simulink model "CAS_MPPT_ESC"  (R2022a)
settings: Solver=VariableStepAuto  StartTime=0.0  StopTime=24  RelTol=1e-12
undefined symbols (not defined in the file or in its folder): sigbuilder_block
settings Model: PacingRate=0.400000  Creator=samso  LastModifiedBy=samso
settings OptimizationCC: BlockReduction=off  DefaultParameterBehavior=Inlined  BufferReuse=off

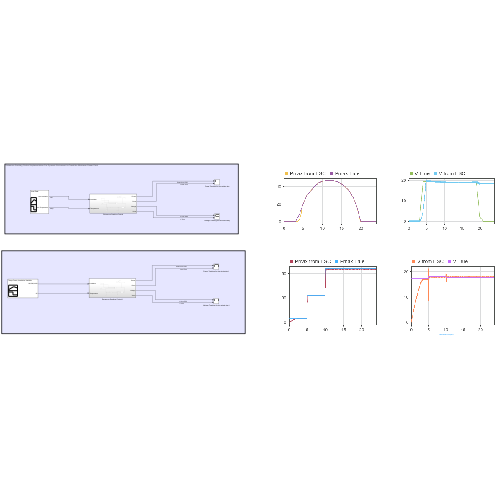
[thumbnail: Simulink's stored preview of the top-level diagram]
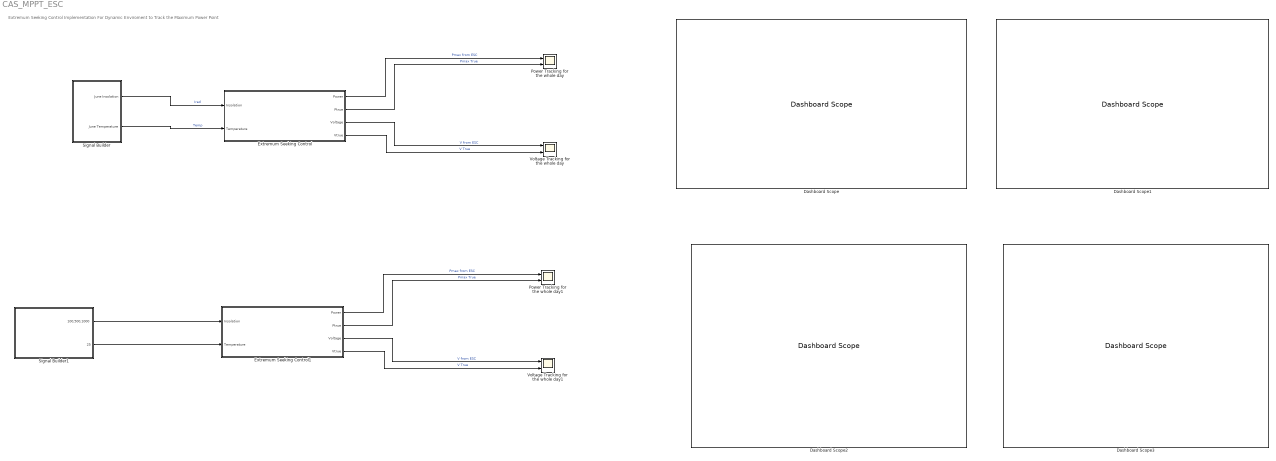
== system CAS_MPPT_ESC ==
  note: Extremum Seeking Control Implementation For Dynamic Enviroment to Track the Maximum Power Point
  Dashboard Scope{,1..3} (4 alike) : DashboardScope
  Extremum Seeking Control : Subsystem
  Extremum Seeking Control1 : Subsystem
  Power Tracking for the whole day : Scope  NumInputPorts=2
  Power Tracking for the whole day1 : Scope  NumInputPorts=2
  Signal Builder : Subsystem  Tag=STV Subsys  LoadFcn=sigbuilder_block('load');  StartFcn=sigbuilder_block('start');  StopFcn=sigbuilder_block('stop');  ClipboardFcn=sigbuilder_block('clipboard');  mask(Sigbuilder block){tuvar=[0:10]}
      mask help: Simulink:masks:SigbuilderBlock_MD
      mask init:
      | if ~strcmp(get_param(bdroot(gcbh),'SimulationStatus'),'stopped') tuvar = sigbuilder_block('maskInit'); end
      settings: CopyFcn=sigbuilder_block('copy');  DeleteFcn=sigbuilder_block('delete');  ModelCloseFcn=sigbuilder_block('modelClose');  PreSaveFcn=sigbuilder_block('preSave');  PauseFcn=sigbuilder_block('pause');  ContinueFcn=sigbuilder_block('continue');  NameChangeFcn=sigbuilder_block('namechange');  OpenFcn=sigbuilder_block('open',[437.25 199.5 386.25 399.75 ]);  CloseFcn=sigbuilder_block('close');
      mask Display: plot(0, 0, 100, 100,[2, 2, 32, 32, 2], [68, 8, 8, 68, 68],[32, 2], [38, 38], [32, 19, 2],[53, 60, 44], [32, 17, 17, 2],[16, 16, 31, 31]);txt = getActiveGroup(gcbh);text(2, 100, txt,'verticalAlignment', 'top');
  Signal Builder1 : Subsystem  Tag=STV Subsys  LoadFcn=sigbuilder_block('load');  StartFcn=sigbuilder_block('start');  StopFcn=sigbuilder_block('stop');  ClipboardFcn=sigbuilder_block('clipboard');  mask(Sigbuilder block){tuvar=[0:10]}
      mask help: Simulink:masks:SigbuilderBlock_MD
      mask init:
      | if ~strcmp(get_param(bdroot(gcbh),'SimulationStatus'),'stopped') tuvar = sigbuilder_block('maskInit'); end
      settings: CopyFcn=sigbuilder_block('copy');  DeleteFcn=sigbuilder_block('delete');  ModelCloseFcn=sigbuilder_block('modelClose');  PreSaveFcn=sigbuilder_block('preSave');  PauseFcn=sigbuilder_block('pause');  ContinueFcn=sigbuilder_block('continue');  NameChangeFcn=sigbuilder_block('namechange');  OpenFcn=sigbuilder_block('open',[0 36 1440 716.25 ]);  CloseFcn=sigbuilder_block('close');
      mask Display: plot(0, 0, 100, 100,[2, 2, 32, 32, 2], [68, 8, 8, 68, 68],[32, 2], [38, 38], [32, 19, 2],[53, 60, 44], [32, 17, 17, 2],[16, 16, 31, 31]);txt = getActiveGroup(gcbh);text(2, 100, txt,'verticalAlignment', 'top');
  Voltage Tracking for the whole day : Scope  NumInputPorts=2
  Voltage Tracking for the whole day1 : Scope  NumInputPorts=2
  wires:
  Extremum Seeking Control/1(Power) -> Power Tracking for the whole day/1  "Pmax from ESC"
  Extremum Seeking Control/2(Ptrue) -> Power Tracking for the whole day/2  "Pmax True"
  Extremum Seeking Control/3(Voltage) -> Voltage Tracking for the whole day/1  "V from ESC"
  Extremum Seeking Control/4(Vtrue) -> Voltage Tracking for the whole day/2  "V True"
  Signal Builder/1(June Insolation) -> Extremum Seeking Control/1(Insolation)  "Irad"
  Signal Builder/2(June Temperature) -> Extremum Seeking Control/2(Temperature)  "Temp"
  Extremum Seeking Control1/3(Voltage) -> Voltage Tracking for the whole day1/1  "V from ESC"
  Extremum Seeking Control1/1(Power) -> Power Tracking for the whole day1/1  "Pmax from ESC"
  Extremum Seeking Control1/4(Vtrue) -> Voltage Tracking for the whole day1/2  "V True"
  Extremum Seeking Control1/2(Ptrue) -> Power Tracking for the whole day1/2  "Pmax True"
  Signal Builder1/1(100,500,1000) -> Extremum Seeking Control1/1(Insolation)
  Signal Builder1/2(25) -> Extremum Seeking Control1/2(Temperature)

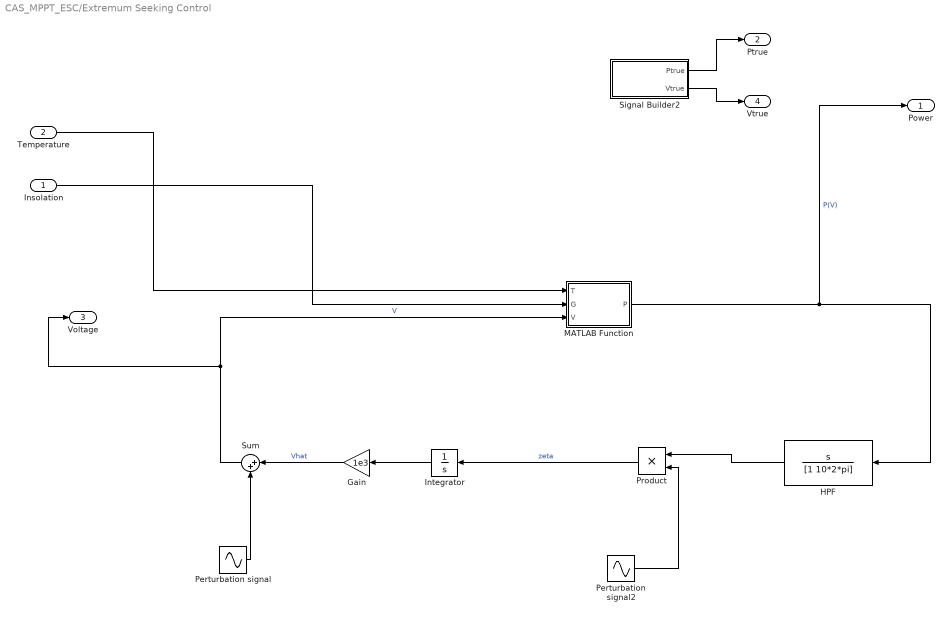
== system CAS_MPPT_ESC/Extremum Seeking Control ==
  Insolation : Inport
  Temperature : Inport  Port=2
  Gain : Gain  Gain=1e3
  HPF : TransferFcn  Numerator=[1 0]  Denominator=[1 10*2*pi]
  Integrator : Integrator
  MATLAB Function : MATLAB Function  TreatAsAtomicUnit=on
  Perturbation signal : Sin  Amplitude=0.2  Frequency=25*2*pi  SampleTime=0
  Perturbation signal2 : Sin  Amplitude=0.2  Frequency=25*2*pi  SampleTime=0
  Product : Product
  Signal Builder2 : Subsystem  Tag=STV Subsys  LoadFcn=sigbuilder_block('load');  StartFcn=sigbuilder_block('start');  StopFcn=sigbuilder_block('stop');  ClipboardFcn=sigbuilder_block('clipboard');  mask(Sigbuilder block){tuvar=[0:10]}
      mask help: Simulink:masks:SigbuilderBlock_MD
      mask init:
      | if ~strcmp(get_param(bdroot(gcbh),'SimulationStatus'),'stopped') tuvar = sigbuilder_block('maskInit'); end
      settings: CopyFcn=sigbuilder_block('copy');  DeleteFcn=sigbuilder_block('delete');  ModelCloseFcn=sigbuilder_block('modelClose');  PreSaveFcn=sigbuilder_block('preSave');  PauseFcn=sigbuilder_block('pause');  ContinueFcn=sigbuilder_block('continue');  NameChangeFcn=sigbuilder_block('namechange');  OpenFcn=sigbuilder_block('open',[6 36 1428 675.75 ]);  CloseFcn=sigbuilder_block('close');
      mask Display: plot(0, 0, 100, 100,[2, 2, 32, 32, 2], [68, 8, 8, 68, 68],[32, 2], [38, 38], [32, 19, 2],[53, 60, 44], [32, 17, 17, 2],[16, 16, 31, 31]);txt = getActiveGroup(gcbh);text(2, 100, txt,'verticalAlignment', 'top');
  Sum : Sum  Inputs=|++
  Power : Outport
  Ptrue : Outport  Port=2
  Voltage : Outport  Port=3
  Vtrue : Outport  Port=4
  wires:
  Product/1 -> Integrator/1  "zeta"
  Perturbation signal/1 -> Sum/2
  Integrator/1 -> Gain/1
  MATLAB Function/1(P) -> Power/1, HPF/1  "P(V)"
  HPF/1 -> Product/1
  Sum/1 -> Voltage/1, MATLAB Function/3(V)  "V"
  Perturbation signal2/1 -> Product/2
  Gain/1 -> Sum/1  "Vhat"
  Insolation/1 -> MATLAB Function/2(G)
  Temperature/1 -> MATLAB Function/1(T)
  Signal Builder2/1(Ptrue) -> Ptrue/1
  Signal Builder2/2(Vtrue) -> Vtrue/1

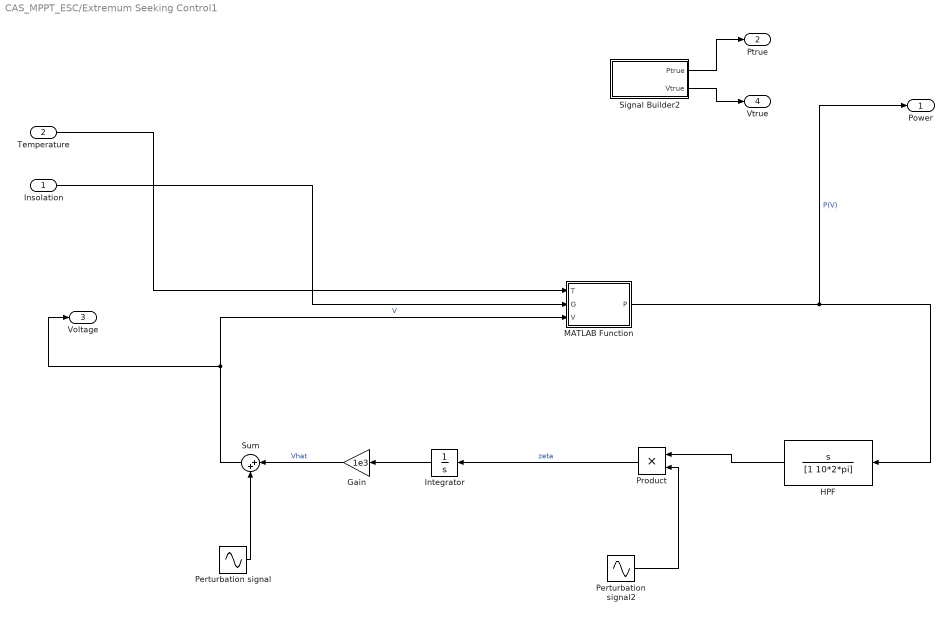
== system CAS_MPPT_ESC/Extremum Seeking Control1 ==
  Insolation : Inport
  Temperature : Inport  Port=2
  Gain : Gain  Gain=1e3
  HPF : TransferFcn  Numerator=[1 0]  Denominator=[1 10*2*pi]
  Integrator : Integrator
  MATLAB Function : MATLAB Function  TreatAsAtomicUnit=on
  Perturbation signal : Sin  Amplitude=0.2  Frequency=25*2*pi  SampleTime=0
  Perturbation signal2 : Sin  Amplitude=0.2  Frequency=25*2*pi  SampleTime=0
  Product : Product
  Signal Builder2 : Subsystem  Tag=STV Subsys  LoadFcn=sigbuilder_block('load');  StartFcn=sigbuilder_block('start');  StopFcn=sigbuilder_block('stop');  ClipboardFcn=sigbuilder_block('clipboard');  mask(Sigbuilder block){tuvar=[0:10]}
      mask help: Simulink:masks:SigbuilderBlock_MD
      mask init:
      | if ~strcmp(get_param(bdroot(gcbh),'SimulationStatus'),'stopped') tuvar = sigbuilder_block('maskInit'); end
      settings: CopyFcn=sigbuilder_block('copy');  DeleteFcn=sigbuilder_block('delete');  ModelCloseFcn=sigbuilder_block('modelClose');  PreSaveFcn=sigbuilder_block('preSave');  PauseFcn=sigbuilder_block('pause');  ContinueFcn=sigbuilder_block('continue');  NameChangeFcn=sigbuilder_block('namechange');  OpenFcn=sigbuilder_block('open',[6 36 1428 675.75 ]);  CloseFcn=sigbuilder_block('close');
      mask Display: plot(0, 0, 100, 100,[2, 2, 32, 32, 2], [68, 8, 8, 68, 68],[32, 2], [38, 38], [32, 19, 2],[53, 60, 44], [32, 17, 17, 2],[16, 16, 31, 31]);txt = getActiveGroup(gcbh);text(2, 100, txt,'verticalAlignment', 'top');
  Sum : Sum  Inputs=|++
  Power : Outport
  Ptrue : Outport  Port=2
  Voltage : Outport  Port=3
  Vtrue : Outport  Port=4
  wires:
  Product/1 -> Integrator/1  "zeta"
  Perturbation signal/1 -> Sum/2
  Integrator/1 -> Gain/1
  MATLAB Function/1(P) -> Power/1, HPF/1  "P(V)"
  HPF/1 -> Product/1
  Sum/1 -> Voltage/1, MATLAB Function/3(V)  "V"
  Perturbation signal2/1 -> Product/2
  Gain/1 -> Sum/1  "Vhat"
  Insolation/1 -> MATLAB Function/2(G)
  Temperature/1 -> MATLAB Function/1(T)
  Signal Builder2/2(Vtrue) -> Vtrue/1
  Signal Builder2/1(Ptrue) -> Ptrue/1

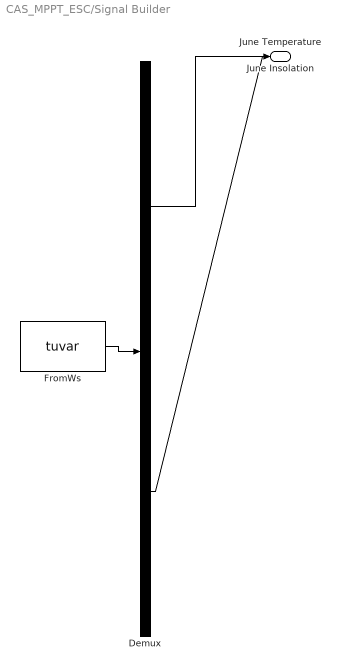
== system CAS_MPPT_ESC/Signal Builder ==
  Demux : Demux  Tag=STV Demux  Outputs=2
      settings: DisplayOption=none
  FromWs : FromWorkspace  Tag=STV FromWs  VariableName=tuvar
      SigBuilderData=|
      | common.afterFinalStr = 'Extrapolate'
      | common.sampleTime = 0
      | dataSet.timeRange = [0 24]
      | dataSet.name = 'June Data'
      | sbobj.Groups.Name = 'June Data'
      | sbobj.Groups.Signals(1).Name = 'June Insolation'
      | sbobj.Groups.Signals(1).XData = [0 1 2 3 4 5 6 7 8 9 10 11 12 13 14 15 16 17 18 19 20 21 22 24]
      | sbobj.Groups.Signals(1).YData = [0 0 0 0 139 297 435 500 576 630 662 676 679 679 657 624 577 509 409 255 5 0 0 0]
      | sbobj.Groups.Signals(2).Name = 'June Temperature'
      | sbobj.Groups.Signals(2).XData = [0 1 2 3 4 5 6 7 8 9 10 11 12 13 14 15 16 17 18 19 20 21 22 23 24]
      | sbobj.Groups.Signals(2).YData = [13.32 12.93 12.69 12.53 12.38 12.52 13.3 14.31 15.22 16.12 16.93 17.62 18.14 18.49 18.67 18.66 18.47 18.08 17.56 16.9 15.89 15 14.28 13.74 13.74]
      | sbobj.Groups.TimeRange = [0 24]
  June Insolation : Outport  Tag=STV Outport
  June Temperature : Outport  Tag=STV Outport  Port=2
  wires:
  FromWs/1 -> Demux/1
  Demux/1 -> June Insolation/1
  Demux/2 -> June Temperature/1

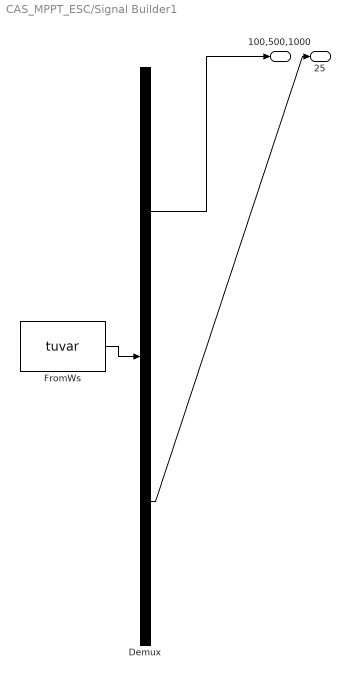
== system CAS_MPPT_ESC/Signal Builder1 ==
  Demux : Demux  Tag=STV Demux  Outputs=2
      settings: DisplayOption=none
  FromWs : FromWorkspace  Tag=STV FromWs  VariableName=tuvar
      SigBuilderData=|
      | common.afterFinalStr = 'Extrapolate'
      | common.sampleTime = 0
      | dataSet.timeRange = [0 24]
      | dataSet.name = 'Temp Const, Insolation Variable'
      | sbobj.Groups.Name = 'Temp Const, Insolation Variable'
      | sbobj.Groups.Signals(1).Name = '100,500,1000'
      | sbobj.Groups.Signals(1).XData = [0 5 5 10 10 24]
      | sbobj.Groups.Signals(1).YData = [100 100 500 500 1000 1000]
      | sbobj.Groups.Signals(2).Name = '25'
      | sbobj.Groups.Signals(2).XData = [0 24]
      | sbobj.Groups.Signals(2).YData = [25 25]
      | sbobj.Groups.TimeRange = [0 24]
  100,500,1000 : Outport  Tag=STV Outport
  25 : Outport  Tag=STV Outport  Port=2
  wires:
  FromWs/1 -> Demux/1
  Demux/1 -> 100,500,1000/1
  Demux/2 -> 25/1

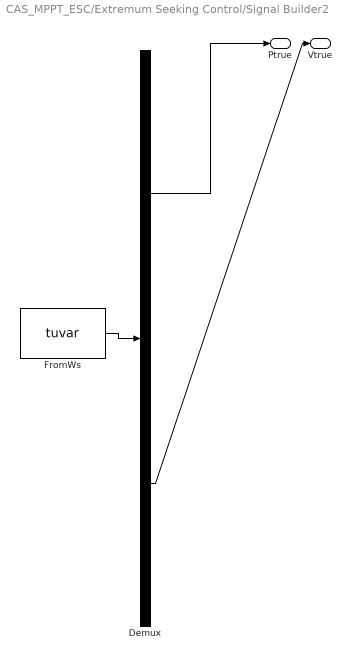
== system CAS_MPPT_ESC/Extremum Seeking Control/Signal Builder2 ==
  Demux : Demux  Tag=STV Demux  Outputs=2
      settings: DisplayOption=none
  FromWs : FromWorkspace  Tag=STV FromWs  VariableName=tuvar
      SigBuilderData=|
      | common.afterFinalStr = 'Extrapolate'
      | common.sampleTime = 0
      | dataSet.timeRange = [0 24]
      | dataSet.name = 'Pmax_true'
      | sbobj.Groups.Name = 'Pmax_true'
      | sbobj.Groups.Signals(1).Name = 'Ptrue'
      | sbobj.Groups.Signals(1).XData = [0 0.1 0.2 0.3 0.4 0.5 0.6 0.7 0.8 0.9 1 1.1 1.2 1.3 1.4 1.5 1.6 1.7 1.8 1.9 2 2.1 2.2 2.3 2.4 2.5 2.6 2.7 2.8 2.9 3 3.1 3.2 3.3 3.4 3.5 3.6 3.7 3.8 3.9 4 4.1 4.2 4.3 4.4 4.5 4.6 4.7 4.8 4.9 5 5.1 5.2 5.3 5.4 5.5 5.6 5.7 5.8 5.9 6 6.1 6.2 6.3 6.4 6.5 6.6 6.7 6.8 6.9 7 7.1 7.2 7.3 7.4 7.5 7.6 7.7 7.8 7.9 8 8.1 8.2 8.3 8.4 8.5 8.6 8.7 8.8 8.9 9 9.1 9.2 9.3 9.4 9.5 9.6 9.7 9.8 9.9 10 10.1 10.2 10.3 10.4 10.5 10.6 10.7 10.8 10.9 11 11.1 11.2 11.3 11.4 11.5 11.6 11.7 11.8 11.9 12 12.1 12.2 12.3 12.4 12.5 12.6 12.7 12.8 12.9 13 13.1 13.2 13.3 13.4 13.5 13.6 13.7 13.8 13.9 14 14.1 14.2 14.3 14.4 14.5 14.6 14.7 14.8 14.9 15 15.1 15.2 15.3 15.4 15.5 15.6 15.7 15.8 15.9 16 16.1 16.2 16.3 16.4 16.5 16.6 16.7 16.8 16.9 17 17.1 17.2 17.3 17.4 17.5 17.6 17.7 17.8 17.9 18 18.1 18.2 18.3 18.4 18.5 18.6 18.7 18.8 18.9 19 19.1 19.2 19.3 19.4 19.5 19.6 19.7 19.8 19.9 20 20.1 20.2 20.3 20.4 20.5 20.6 20.7 20.8 20.9 21 21.1 21.2 21.3 21.4 21.5 21.6 21.7 21.8 21.9 22 22.1 22.2 22.3 22.4 22.5 22.6 22.7 22.8 22.9 23 23.1 23.2 23.3 23.4 23.5 23.6 23.7 23.8 23.9 24]
      | sbobj.Groups.Signals(1).YData = [0 0 0 0 0 0 0 0 0 0 0 0 ... (241 elements, 1x241)]
      | sbobj.Groups.Signals(2).Name = 'Vtrue'
      | sbobj.Groups.Signals(2).XData = [0 0.1 0.2 0.3 0.4 0.5 0.6 0.7 0.8 0.9 1 1.1 1.2 1.3 1.4 1.5 1.6 1.7 1.8 1.9 2 2.1 2.2 2.3 2.4 2.5 2.6 2.7 2.8 2.9 3 3.1 3.2 3.3 3.4 3.5 3.6 3.7 3.8 3.9 4 4.1 4.2 4.3 4.4 4.5 4.6 4.7 4.8 4.9 5 5.1 5.2 5.3 5.4 5.5 5.6 5.7 5.8 5.9 6 6.1 6.2 6.3 6.4 6.5 6.6 6.7 6.8 6.9 7 7.1 7.2 7.3 7.4 7.5 7.6 7.7 7.8 7.9 8 8.1 8.2 8.3 8.4 8.5 8.6 8.7 8.8 8.9 9 9.1 9.2 9.3 9.4 9.5 9.6 9.7 9.8 9.9 10 10.1 10.2 10.3 10.4 10.5 10.6 10.7 10.8 10.9 11 11.1 11.2 11.3 11.4 11.5 11.6 11.7 11.8 11.9 12 12.1 12.2 12.3 12.4 12.5 12.6 12.7 12.8 12.9 13 13.1 13.2 13.3 13.4 13.5 13.6 13.7 13.8 13.9 14 14.1 14.2 14.3 14.4 14.5 14.6 14.7 14.8 14.9 15 15.1 15.2 15.3 15.4 15.5 15.6 15.7 15.8 15.9 16 16.1 16.2 16.3 16.4 16.5 16.6 16.7 16.8 16.9 17 17.1 17.2 17.3 17.4 17.5 17.6 17.7 17.8 17.9 18 18.1 18.2 18.3 18.4 18.5 18.6 18.7 18.8 18.9 19 19.1 19.2 19.3 19.4 19.5 19.6 19.7 19.8 19.9 20 20.1 20.2 20.3 20.4 20.5 20.6 20.7 20.8 20.9 21 21.1 21.2 21.3 21.4 21.5 21.6 21.7 21.8 21.9 22 22.1 22.2 22.3 22.4 22.5 22.6 22.7 22.8 22.9 23 23.1 23.2 23.3 23.4 23.5 23.6 23.7 23.8 23.9 24]
      | sbobj.Groups.Signals(2).YData = [0 0 0 0 0 0 0 0 0 0 0 0 ... (241 elements, 1x241)]
      | sbobj.Groups.TimeRange = [0 24]
  Ptrue : Outport  Tag=STV Outport
  Vtrue : Outport  Tag=STV Outport  Port=2
  wires:
  FromWs/1 -> Demux/1
  Demux/1 -> Ptrue/1
  Demux/2 -> Vtrue/1

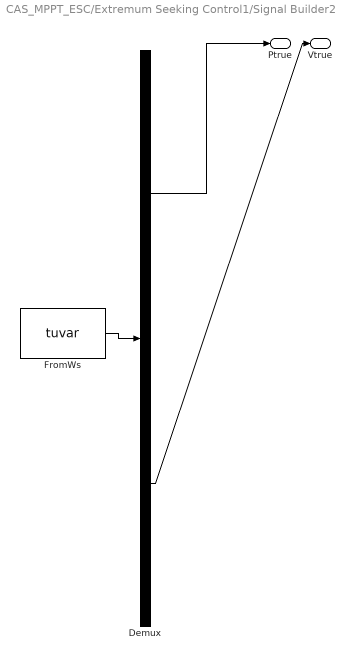
== system CAS_MPPT_ESC/Extremum Seeking Control1/Signal Builder2 ==
  Demux : Demux  Tag=STV Demux  Outputs=2
      settings: DisplayOption=none
  FromWs : FromWorkspace  Tag=STV FromWs  VariableName=tuvar
      SigBuilderData=|
      | common.afterFinalStr = 'Extrapolate'
      | common.sampleTime = 0
      | dataSet.timeRange = [0 24]
      | dataSet.name = 'Pmax_true'
      | sbobj.Groups.Name = 'Pmax_true'
      | sbobj.Groups.Signals(1).Name = 'Ptrue'
      | sbobj.Groups.Signals(1).XData = [0 5 5 10 10 14.4 15 24]
      | sbobj.Groups.Signals(1).YData = [5.1088 5.1088 32.6025 32.6025 65.5 65.5 65.5 65.5]
      | sbobj.Groups.Signals(2).Name = 'Vtrue'
      | sbobj.Groups.Signals(2).XData = [0 5 5 10 10 12 24]
      | sbobj.Groups.Signals(2).YData = [17.017 17.017 17.901 17.901 17.68 17.68 17.68]
      | sbobj.Groups.TimeRange = [0 24]
  Ptrue : Outport  Tag=STV Outport
  Vtrue : Outport  Tag=STV Outport  Port=2
  wires:
  FromWs/1 -> Demux/1
  Demux/1 -> Ptrue/1
  Demux/2 -> Vtrue/1

== matlab function CAS_MPPT_ESC/Extremum Seeking Control/MATLAB Function ==
  data: T input; P output; G input; V input
function P = PV_obj_function(T,G,V)
ai=0.034/100;                     % Current Tmperature coefficient(ki)
av=-0.34/100;                     % Voltage Tmperature coefficient(kv)
Isc_r=3.99;                        % Short-circuit current
Voc_r=22.1;                       % Opent circuit voltage
Vm=17.6;                            % Maximum voltage @ STC
Im=3.69;                          % Maximum current @ STC
Pm=65;                           % Maximum power   @ STC
Ns=36;                            % nomber of Cells   
n=0.9;                            % Diode ideality factor

%% Internal parameters%%%%%%%%%%%%%
Gr=1000;                          % reference irradiance
T=T+273.6;                        % 
Tr= 25 +273.6;                    % Temperature reference
dT=T-Tr;
Isc=Isc_r+ai*dT;                  % variation of Isc with T°
Voc=Voc_r+av*dT;                  % variation de Vco with T°
q=1.60217646*power(10,-19);       % charge constant
K=1.3806503*power(10,-23);        % Boltzmann constant
Vt=(Ns*n*K*T/q);                  % Thermal voltage 
Eg=1.12;                          % gap energy
Iph=Isc*(G/Gr);                   % photo-current
Iss=(Isc)/(   exp( Voc/Vt )-1 );  % saturation current
Is=Iss*( (T/Tr)^3 ) * exp ( ( (q*Eg)/(n*K) )*((1/Tr)-(1/T)) );%saturation current
Rs=0.5;                           % series resistance 
Rp=195;                           % parallele resistance
%%
I=Iph;             % initial codition

    
        
    for n2=1:20                          % Newton-Raphson loop for calculating output current
    Vd= (V+Rs*I);                    % Diode Voltage
    Id=Is*( exp(Vd/Vt) -1);              % Diode current
    Ip=Vd/Rp;                            % Parallele resistance Current
    f=Iph-I-Id-Ip;                       % f(I)=0
    df=-1-(Is*Rs/Vt)*exp(Vd/Vt)-(Rs/Rp); % f'(I)=0
    I=I-f/df;% Newton-Raphson formula
    
    end % end of Newton-Raphson
    
    if I<0
        I=0;
    end
    Ipv=I;                           % Accumulation of output currant 
%%
 
P=Ipv.*V; end

== matlab function CAS_MPPT_ESC/Extremum Seeking Control1/MATLAB Function ==
  data: T input; P output; G input; V input
function P = PV_obj_function(T,G,V)
ai=0.034/100;                     % Current Tmperature coefficient(ki)
av=-0.34/100;                     % Voltage Tmperature coefficient(kv)
Isc_r=3.99;                        % Short-circuit current
Voc_r=22.1;                       % Opent circuit voltage
Vm=17.6;                            % Maximum voltage @ STC
Im=3.69;                          % Maximum current @ STC
Pm=65;                           % Maximum power   @ STC
Ns=36;                            % nomber of Cells   
n=0.9;                            % Diode ideality factor

%% Internal parameters%%%%%%%%%%%%%
Gr=1000;                          % reference irradiance
T=T+273.6;                        % 
Tr= 25 +273.6;                    % Temperature reference
dT=T-Tr;
Isc=Isc_r+ai*dT;                  % variation of Isc with T°
Voc=Voc_r+av*dT;                  % variation de Vco with T°
q=1.60217646*power(10,-19);       % charge constant
K=1.3806503*power(10,-23);        % Boltzmann constant
Vt=(Ns*n*K*T/q);                  % Thermal voltage 
Eg=1.12;                          % gap energy
Iph=Isc*(G/Gr);                   % photo-current
Iss=(Isc)/(   exp( Voc/Vt )-1 );  % saturation current
Is=Iss*( (T/Tr)^3 ) * exp ( ( (q*Eg)/(n*K) )*((1/Tr)-(1/T)) );%saturation current
Rs=0.5;                           % series resistance 
Rp=195;                           % parallele resistance
%%
I=Iph;             % initial codition

    
        
    for n2=1:20                          % Newton-Raphson loop for calculating output current
    Vd= (V+Rs*I);                    % Diode Voltage
    Id=Is*( exp(Vd/Vt) -1);              % Diode current
    Ip=Vd/Rp;                            % Parallele resistance Current
    f=Iph-I-Id-Ip;                       % f(I)=0
    df=-1-(Is*Rs/Vt)*exp(Vd/Vt)-(Rs/Rp); % f'(I)=0
    I=I-f/df;% Newton-Raphson formula
    
    end % end of Newton-Raphson
    
    if I<0
        I=0;
    end
    Ipv=I;                           % Accumulation of output currant 
%%
 
P=Ipv.*V; end
